simulink model "Maglev_3"  (R2016b)
settings: Solver=VariableStepAuto  StartTime=0.0  StopTime=10.0  RelTol=1e-3
values from neighbouring files (symbols this model uses):
  g = 9.81    [Maglev_2.m]
  Kad = 0.2    [Maglev_2.m]
  Kam = 100    [Maglev_2.m]
  Kda = 10    [Maglev_2.m]
  Kdl = 34    [Maglev_2.m]
  Kel = 33e4    (= 330000)    [Maglev_2.m]
  Kf = 0.653e-6    (= 6.53e-07)    [Maglev_2.m]
  Kfv = 0.02    [Maglev_2.m]
  Ks = 13.33    [Maglev_2.m]
  Kx = 10    [Maglev_2.m]
  L = 6.3e-3    (= 0.0063)    [Maglev_2.m]
  Lc = 0.03    [Maglev_2.m]
  mk = 8.37e-3    (= 0.00837)    [Maglev_2.m]
  Rc = 3.5    [Maglev_2.m]
  Rs = 0.25    [Maglev_2.m]
  u0 = 0    [Maglev_2.m]
  x0 = 9.02e-3    (= 0.00902)    [Maglev_2.m]
  y0 = 0.054    [Maglev_2.m]
  ymu0 = 0    [Maglev_2.m]
undefined symbols (not defined in the file or in its folder): sigbuilder_block
libraries: simulink x1
settings Model: Creator=Niels  LastModifiedBy=Niels

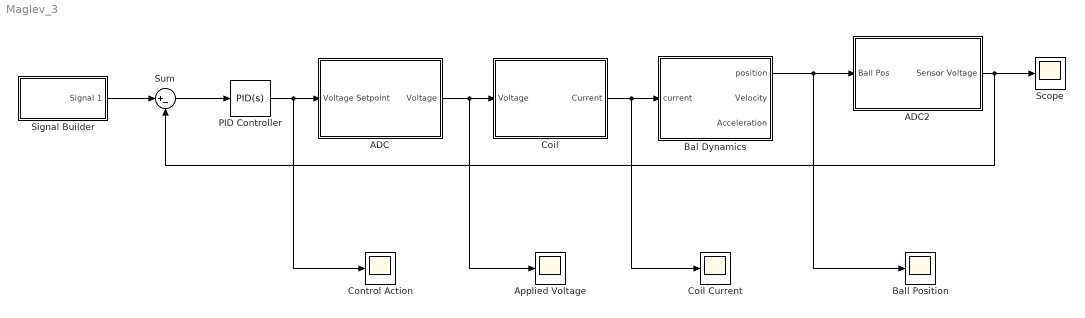
== system Maglev_3 ==
  ADC : Subsystem
  "ADC2 " : Subsystem
  Applied Voltage : Scope
  Bal Dynamics : Subsystem
  Ball Position : Scope
  Coil : Subsystem
  Coil Current : Scope
  Control Action : Scope
  PID Controller : simulink/Continuous/PID Controller  Controller=PID  TimeDomain=Continuous-time  SampleTime=-1  IntegratorMethod=Forward Euler  FilterMethod=Forward Euler  Form=Ideal  UseFilter=on  ControllerParametersSource=internal  P=3.5  I=1  D=0.001  N=100  InitialConditionSource=internal  InitialConditionForIntegrator=0  InitialConditionForFilter=0  ExternalReset=none  LimitOutput=on  UpperSaturationLimit=1  LowerSaturationLimit=0  LinearizeAsGain=on  AntiWindupMode=none  Kb=1  TrackingMode=off  Kt=1  PParamMin=[]  PParamMax=[]  IParamMin=[]  IParamMax=[]  DParamMin=[]  DParamMax=[]  NParamMin=[]  NParamMax=[]  KbParamMin=[]  KbParamMax=[]  KtParamMin=[]  KtParamMax=[]  POutMin=[]  POutMax=[]  IOutMin=[]  IOutMax=[]  DOutMin=[]  DOutMax=[]  NOutMin=[]  NOutMax=[]  KbOutMin=[]  KbOutMax=[]  KtOutMin=[]  KtOutMax=[]  IntegratorOutMin=[]  IntegratorOutMax=[]  FilterOutMin=[]  FilterOutMax=[]  SumOutMin=[]  SumOutMax=[]  SumI1OutMin=[]  SumI1OutMax=[]  SumI2OutMin=[]  SumI2OutMax=[]  SumI3OutMin=[]  SumI3OutMax=[]  SumDOutMin=[]  SumDOutMax=[]  SaturationOutMin=[]  SaturationOutMax=[]  IntegratorContinuousStateAttributes=''  IntegratorStateMustResolveToSignalObject=off  IntegratorRTWStateStorageClass=Auto  FilterContinuousStateAttributes=''  FilterStateMustResolveToSignalObject=off  FilterRTWStateStorageClass=Auto  DifferentiatorICPrevScaledInput=0  DifferentiatorOutMin=[]  DifferentiatorOutMax=[]
  Scope : Scope
  Signal Builder : Subsystem  Tag=STV Subsys  LoadFcn=sigbuilder_block('load');  StartFcn=sigbuilder_block('start');  StopFcn=sigbuilder_block('stop');  ClipboardFcn=sigbuilder_block('clipboard');  mask(Sigbuilder block){tuvar=[0:10]}
      mask help: Simulink:masks:SigbuilderBlock_MD
      mask init:
      | if ~strcmp(get_param(bdroot(gcbh),'SimulationStatus'),'stopped') tuvar = sigbuilder_block('maskInit'); end
      settings: CopyFcn=sigbuilder_block('copy');  DeleteFcn=sigbuilder_block('delete');  ModelCloseFcn=sigbuilder_block('modelClose');  PreSaveFcn=sigbuilder_block('preSave');  PauseFcn=sigbuilder_block('pause');  ContinueFcn=sigbuilder_block('continue');  NameChangeFcn=sigbuilder_block('namechange');  OpenFcn=sigbuilder_block('open',[437.6 199.2 550.4 400 ]);  CloseFcn=sigbuilder_block('close');
      mask Display: plot(0, 0, 100, 100,[2, 2, 32, 32, 2], [68, 8, 8, 68, 68],[32, 2], [38, 38], [32, 19, 2],[53, 60, 44], [32, 17, 17, 2],[16, 16, 31, 31]);txt = getActiveGroup(gcbh);text(2, 100, txt,'verticalAlignment', 'top');
  Sum : Sum  Inputs=|+-
  wires:
  ADC/1(Voltage) -> Applied Voltage/1, Coil/1("Voltage ")
  Coil/1(Current) -> Coil Current/1, Bal Dynamics/1(current)
  Bal Dynamics/1("position ") -> Ball Position/1, "ADC2 "/1("Ball Pos ")
  PID Controller/1 -> Control Action/1, ADC/1(Voltage Setpoint)
  Sum/1 -> PID Controller/1
  Signal Builder/1(Signal 1) -> Sum/1
  "ADC2 "/1("Sensor Voltage ") -> Scope/1, Sum/2

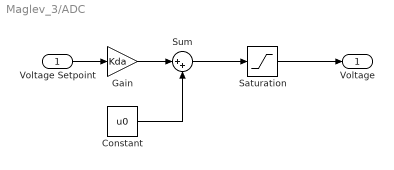
== system Maglev_3/ADC ==
  Voltage Setpoint : Inport
  Constant : Constant  Value=u0
  Gain : Gain  Gain=Kda
  Saturation : Saturate  UpperLimit=5  LowerLimit=0
  Sum : Sum  Inputs=|++
  Voltage : Outport
  wires:
  Voltage Setpoint/1 -> Gain/1
  Sum/1 -> Saturation/1
  Saturation/1 -> Voltage/1
  Gain/1 -> Sum/1
  Constant/1 -> Sum/2

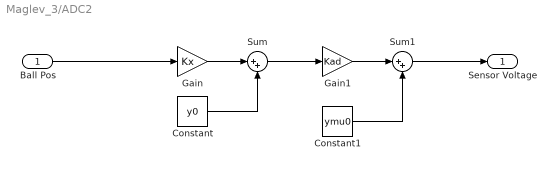
== system Maglev_3/ADC2  ==
  "Ball Pos " : Inport
  Constant : Constant  Value=y0
  Constant1 : Constant  Value=ymu0
  Gain : Gain  Gain=Kx
  Gain1 : Gain  Gain=Kad
  Sum : Sum  Inputs=|++
  Sum1 : Sum  Inputs=|++
  "Sensor Voltage " : Outport
  wires:
  Sum1/1 -> "Sensor Voltage "/1
  Constant/1 -> Sum/2
  "Ball Pos "/1 -> Gain/1
  Sum/1 -> Gain1/1
  Gain1/1 -> Sum1/1
  Gain/1 -> Sum/1
  Constant1/1 -> Sum1/2

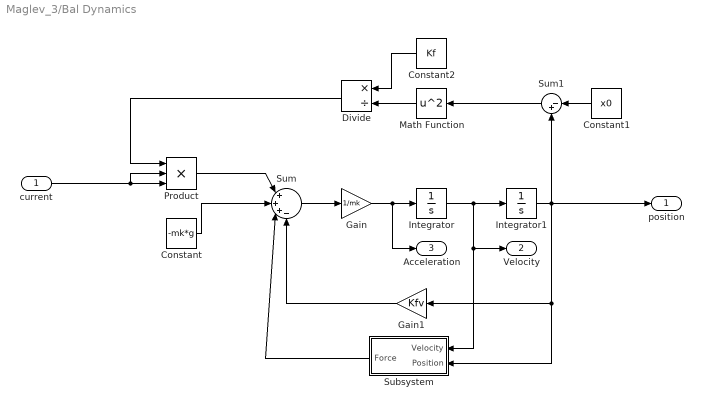
== system Maglev_3/Bal Dynamics ==
  current : Inport
  Constant : Constant  Value=-mk*g
  Constant1 : Constant  Value=x0
  Constant2 : Constant  Value=Kf
  Divide : Product  Inputs=*/
  Gain : Gain  Gain=1/mk
  Gain1 : Gain  Gain=Kfv
  Integrator : Integrator
  Integrator1 : Integrator  LimitOutput=on  UpperSaturationLimit=L  LowerSaturationLimit=0
  Math Function : Math  Operator=square  SaturateOnIntegerOverflow=on
  Product : Product  Inputs=3
  Subsystem : Subsystem
  Sum : Sum  Inputs=|+++-
  Sum1 : Sum  Inputs=|-+
  "position " : Outport
  Velocity : Outport  Port=2
  Acceleration : Outport  Port=3
  wires:
  Sum/1 -> Gain/1
  Product/1 -> Sum/1
  current/1 -> Product/2, Product/3
  Sum1/1 -> Math Function/1
  Integrator/1 -> Subsystem/1(Velocity), Velocity/1, Integrator1/1
  Gain/1 -> Acceleration/1, Integrator/1
  Divide/1 -> Product/1
  Constant1/1 -> Sum1/1
  Integrator1/1 -> Subsystem/2(Position), Gain1/1, "position "/1, Sum1/2
  Constant/1 -> Sum/2
  Constant2/1 -> Divide/1
  Math Function/1 -> Divide/2
  Gain1/1 -> Sum/4
  Subsystem/1(Force) -> Sum/3

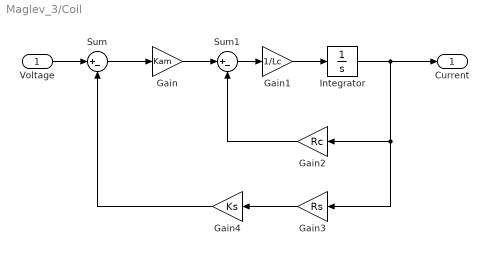
== system Maglev_3/Coil ==
  "Voltage " : Inport
  Gain : Gain  Gain=Kam
  Gain1 : Gain  Gain=1/Lc
  Gain2 : Gain  Gain=Rc
  Gain3 : Gain  Gain=Rs
  Gain4 : Gain  Gain=Ks
  Integrator : Integrator
  Sum : Sum  Inputs=|+-
  Sum1 : Sum  Inputs=|+-
  Current : Outport
  wires:
  Gain/1 -> Sum1/1
  Sum/1 -> Gain/1
  Sum1/1 -> Gain1/1
  "Voltage "/1 -> Sum/1
  Gain3/1 -> Gain4/1
  Gain1/1 -> Integrator/1
  Integrator/1 -> Current/1, Gain3/1, Gain2/1
  Gain4/1 -> Sum/2
  Gain2/1 -> Sum1/2

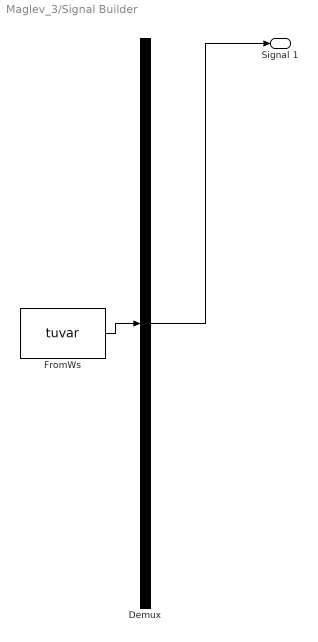
== system Maglev_3/Signal Builder ==
  Demux : Demux  Tag=STV Demux  Outputs=1
  FromWs : FromWorkspace  Tag=STV FromWs  VariableName=tuvar  SampleTime=0
      SigBuilderData=|
      | common.afterFinalStr = 'Extrapolate'
      | common.sampleTime = 0
      | dataSet.timeRange = [0 10]
      | dataSet.name = 'Group 1'
      | sbobj.Groups.Name = 'Group 1'
      | sbobj.Groups.Signals.Name = 'Signal 1'
      | sbobj.Groups.Signals.XData = [0 1.12 1.12 10]
      | sbobj.Groups.Signals.YData = [0 0 0.375 0.375]
  Signal 1 : Outport  Tag=STV Outport
  wires:
  Demux/1 -> Signal 1/1
  FromWs/1 -> Demux/1

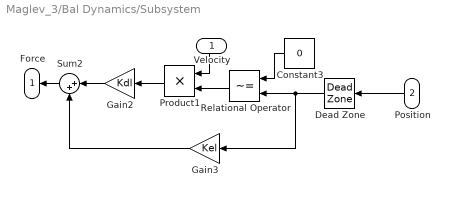
== system Maglev_3/Bal Dynamics/Subsystem ==
  Velocity : Inport
  Position : Inport  Port=2
  Constant3 : Constant  Value=0
  Dead Zone : DeadZone  LowerValue=0  UpperValue=L  SaturateOnIntegerOverflow=on
  Gain2 : Gain  Gain=Kdl
  Gain3 : Gain  Gain=Kel
  Product1 : Product
  Relational Operator : RelationalOperator  Operator=~=  OutDataTypeStr=boolean  RndMeth=Simplest
  Sum2 : Sum  Inputs=|++
  Force : Outport
  wires:
  Dead Zone/1 -> Gain3/1, Relational Operator/2
  Position/1 -> Dead Zone/1
  Velocity/1 -> Product1/1
  Constant3/1 -> Relational Operator/1
  Gain2/1 -> Sum2/1
  Gain3/1 -> Sum2/2
  Sum2/1 -> Force/1
  Product1/1 -> Gain2/1
  Relational Operator/1 -> Product1/2
